simulink model "PROBLEM4"  (R2020b)
settings: Solver=VariableStepAuto  StartTime=0.0  StopTime=10.0  RelTol=1e-3
values from neighbouring files (symbols this model uses):
  b = 3.5077E-6    [datadic.sldd]
  J = 3.2284E-6    [datadic.sldd]
  L = 2.75E-6    [datadic.sldd]
  R = 4.0    [datadic.sldd]
undefined symbols (not defined in the file or in its folder): Kd, Ke, Ki, Kp, Kt
settings Model: Creator=ARPITA  LastModifiedBy=ARPITA

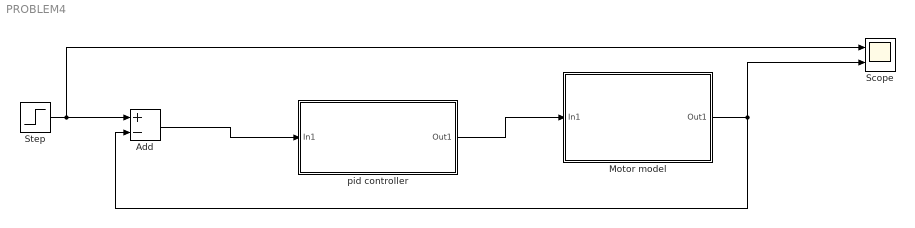
== system PROBLEM4 ==
  Add : Sum  Inputs=+-
  Motor model : Subsystem
  Scope : Scope  NumInputPorts=2
  Step : Step  After=230  SampleTime=0
  pid controller : Subsystem
  wires:
  Motor model/1(Out1) -> Add/2, Scope/2
  pid controller/1(Out1) -> Motor model/1(In1)
  Step/1 -> Scope/1, Add/1
  Add/1 -> pid controller/1(In1)

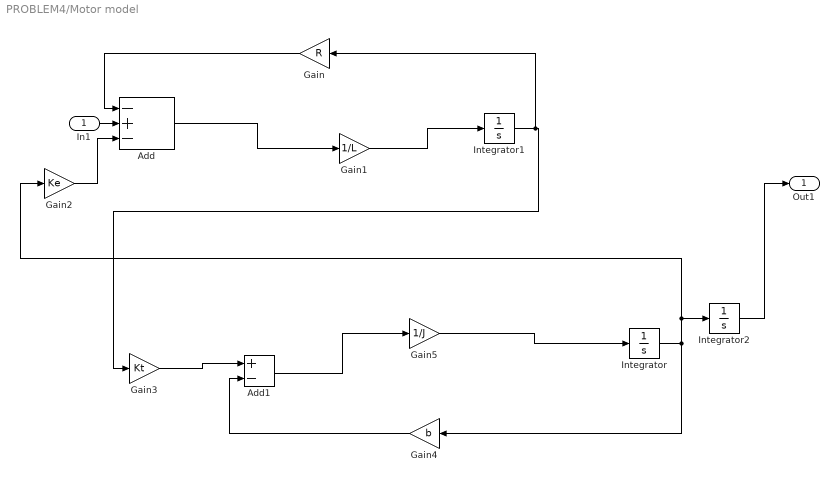
== system PROBLEM4/Motor model ==
  In1 : Inport
  Add : Sum  Inputs=-+-
  Add1 : Sum  Inputs=+-
  Gain : Gain  Gain=R
  Gain1 : Gain  Gain=1/L
  Gain2 : Gain  Gain=Ke
  Gain3 : Gain  Gain=Kt
  Gain4 : Gain  Gain=b
  Gain5 : Gain  Gain=1/J
  Integrator : Integrator
  Integrator1 : Integrator
  Integrator2 : Integrator
  Out1 : Outport
  wires:
  Gain4/1 -> Add1/2
  Integrator2/1 -> Out1/1
  Add/1 -> Gain1/1
  Integrator/1 -> Gain2/1, Integrator2/1, Gain4/1
  Gain1/1 -> Integrator1/1
  Gain5/1 -> Integrator/1
  Gain2/1 -> Add/3
  Integrator1/1 -> Gain/1, Gain3/1
  In1/1 -> Add/2
  Gain/1 -> Add/1
  Add1/1 -> Gain5/1
  Gain3/1 -> Add1/1

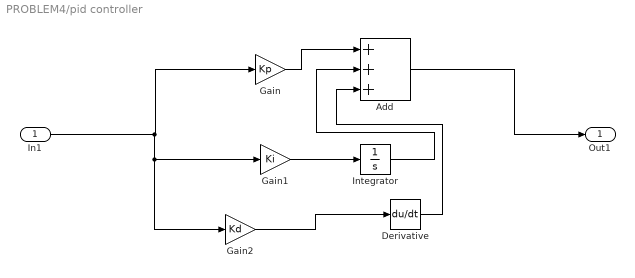
== system PROBLEM4/pid controller ==
  In1 : Inport
  Add : Sum  Inputs=+++
  Derivative : Derivative
  Gain : Gain  Gain=Kp
  Gain1 : Gain  Gain=Ki
  Gain2 : Gain  Gain=Kd
  Integrator : Integrator
  Out1 : Outport
  wires:
  Gain1/1 -> Integrator/1
  Gain/1 -> Add/1
  In1/1 -> Gain1/1, Gain2/1, Gain/1
  Add/1 -> Out1/1
  Gain2/1 -> Derivative/1
  Integrator/1 -> Add/2
  Derivative/1 -> Add/3
